simulink model "IIR_filter"  (R2019a)
settings: Solver=FixedStepAuto  StartTime=0.0  StopTime=10.0  FixedStep=1  RelTol=1e-3
model workspace (MAT data in the model file):
  a1 = 0.5
  a2 = -0.25
  b0 = 1
  b1 = 0.4
settings Model: Creator=rutvi  LastModifiedBy=rutvi
settings DataIOCC: SaveOutput=off  SaveTime=off

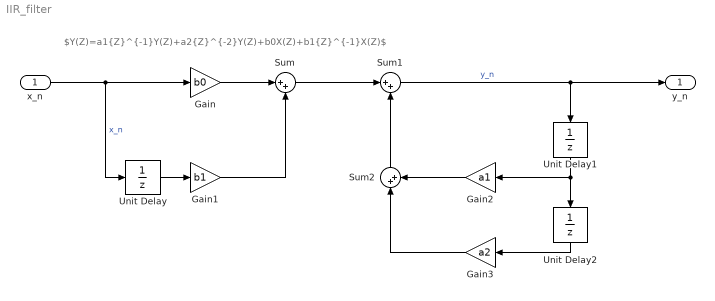
== system IIR_filter ==
  note: $Y(Z)=a1{Z}^{-1}Y(Z)+a2{Z}^{-2}Y(Z)+b0X(Z)+b1{Z}^{-1}X(Z)$
  x_n : Inport  OutDataTypeStr=double  PortDimensions=1  SampleTime=[1,0]
  Gain : Gain  Gain=b0
  Gain1 : Gain  Gain=b1
  Gain2 : Gain  Gain=a1
  Gain3 : Gain  Gain=a2
  Sum : Sum  Inputs=|++
  Sum1 : Sum  Inputs=|++
  Sum2 : Sum  Inputs=|++
  Unit Delay : UnitDelay  SampleTime=-1  HasFrameUpgradeWarning=on
  Unit Delay1 : UnitDelay  SampleTime=-1  HasFrameUpgradeWarning=on
  Unit Delay2 : UnitDelay  SampleTime=-1  HasFrameUpgradeWarning=on
  y_n : Outport  OutDataTypeStr=double  PortDimensions=1  SampleTime=[1,0]
  wires:
  Gain1/1 -> Sum/2
  x_n/1 -> Gain/1, Unit Delay/1  "x_n"
  Gain/1 -> Sum/1
  Unit Delay/1 -> Gain1/1
  Unit Delay1/1 -> Gain2/1, Unit Delay2/1
  Gain3/1 -> Sum2/1
  Sum1/1 -> Unit Delay1/1, y_n/1  "y_n"
  Gain2/1 -> Sum2/2
  Unit Delay2/1 -> Gain3/1
  Sum/1 -> Sum1/1
  Sum2/1 -> Sum1/2
